simulink model "Traffic_Light_cs - 原始版本留存"  (R2020a)
settings: Solver=ode5  StartTime=0.0  StopTime=200  FixedStep=1/1000  RelTol=1e-3
PreLoadFcn:
  | mbxruntime.callbacks.PreLoadFcn(bdroot);
PostLoadFcn:
  | mbxruntime.callbacks.PostLoadFcn(bdroot);
InitFcn:
  | mbxruntime.callbacks.InitFcn(bdroot);
StartFcn:
  | mbxruntime.callbacks.StartFcn(bdroot);
StopFcn:
  | mbxruntime.callbacks.StopFcn(bdroot);
model workspace (MAT data in the model file):
  mbox_table : object (value not decoded)
  model_closed = 0
  sim_status = 0
values from neighbouring files (symbols this model uses):
  q_pass = [0 0 0 37.0489514481 49.8894252687 51.0913174965 61.791576133 65.4762304223 75.669686677 80.4628164105 88.6197377629 94.2384891559 ... (437675 elements, 87535x5)]    [Data_ckx.mat]
  q_stop = [0 0 0 15.0544571491 15.7911831418 16.0935138936 18.6666396431 19.4721381181 21.7098800606 22.5642135149 25.0883481215 26.1253405703 ... (437675 elements, 87535x5)]    [Data_ckx.mat]
  s = roadinf.s    [Constraint_T_V.m]    (also in Light_Distinguish_old.m = 75:-0.7:75-84*0.7)
undefined symbols (not defined in the file or in its folder): InitImageOutputDir, mbxruntime, sigbuilder_block, tabledata
libraries: simulink x10, PreScanSimulinkLibrary x8, simulink_extras x4, autolibshared x1, fuzblock x1
(part 5 of 5)

== matlab function Traffic_Light_cs - 原始版本留存/CAR_Ahead/Decision/Function-Call Subsystem/Subsystem/MATLAB Function ==
  data: Dis input; R_Ori input; Light_State output; G_Ori input; B_Ori input
function Light_State = Light_Distinguish(Dis,R_Ori,G_Ori,B_Ori)

Image=zeros(1800,1920,3);

Image(:,:,1)=R_Ori;
Image(:,:,2)=G_Ori;
Image(:,:,3)=B_Ori;

Light_State=-1;

if Dis>=75
    Light_State=-1;
else
    %%
    
    Gray=rgb2gray(Image);
    
    R=Image(:,:,1); G=Image(:,:,2); B=Image(:,:,3);
    % figure(1),
    % subplot(2,2,1),imshow(Image),title('image')
    % subplot(2,2,2),imshow(R),title('r')
    % subplot(2,2,3),imshow(G),title('g')
    % subplot(2,2,4),imshow(B),title('b')
    
    diff_R=80; diff_G=30; diff_B=10;  % 设置红、绿、蓝三种颜色提取阈值（越大越严格）
    s=75:-0.7:75-84*0.7;
    yy=[765 762 760 759 758 756 755 753 751 750 748 746 744 743 742 740 738 737 734 732 731 729 ...
     727 725 722 720 718 716 712 711 707 705 702 700 695 694 690 687 682 680 678 671 670 666 ...
     663 656 653 650 646 640 636 631 627 621 616 608 602 597 592 587 577 570 562 551 544 536 528 ...
     516 505 495 483 473 459 443 429 413 395 379 358 336 312 289 262 242 202];
    p=polyfit(s,yy,5);
    start=ceil(polyval(p,Dis));
    start=max(start-50,1);     %搜索窗上限
    %%
    % 红色提取
    
    Image_R=Image;
    
    RP_R=Image(:,:,1); RP_G=Image(:,:,2); RP_B=Image(:,:,3);
    
    % figure(2),
    % subplot(2,2,1),imshow(Image),title('image')
    % subplot(2,2,2),imshow(RP_R),title('RP_Rr')
    % subplot(2,2,3),imshow(RP_G),title('RP_Gg')
    % subplot(2,2,4),imshow(RP_B),title('RP_Bb')
    
    XYR=~((R-G)>diff_R&(R-B)>diff_R);  % 提取红色条件是R分量与G、B分量差值大于设定
    
    Mask=Gray(XYR);  % 灰照片掩膜
    
    RP_R(XYR)=Mask; RP_G(XYR)=Mask; RP_B(XYR)=Mask;  % 使得非红色区域变为灰色
    
    Image_R(:,:,1)=RP_R; Image_R(:,:,2)=RP_G; Image_R(:,:,3)=RP_B;
    if start<=300
        start=310;
    end
    SearchRangeR=XYR(start-300:start+200,700:1240);   %确定搜索范围
    if length(find((SearchRangeR)==0))>=1
        Light_State=1;
    end
    
    %%
    % 绿色提取
    Image_G=Image;
    
    GP_R=Image(:,:,1); GP_G=Image(:,:,2); GP_B=Image(:,:,3);
    
    XYG=~((G-R)>diff_G&(G-B)>diff_G);  % 提取绿色条件是G分量与R、B分量差值大于设定
    
    % Mask=Gray(XYG);  % 灰照片掩膜
    Mask=0;
    
    GP_R(XYG)=Mask; GP_G(XYG)=Mask; GP_B(XYG)=Mask;  % 使得非绿色区域变为灰色
    
    Image_G(:,:,1)=GP_R; Image_G(:,:,2)=GP_G; Image_G(:,:,3)=GP_B;
    
    if start<=100
        start=110;
    end
    SearchRangeG=XYG(start-100:start+200,500:1420);   %确定搜索范围
    
    if length(find((SearchRangeG)==0))>=50
        Light_State=2;
    end
    
    %%
    % 蓝色提取
    
    Image_B=Image;
    
    BP_R=Image(:,:,1);BP_G=Image(:,:,2);BP_B=Image(:,:,3);
    
    XYB=~((B-R)>diff_B&(B-G)>diff_B);  % 提取绿色条件是G分量与R、B分量差值大于设定
    
    Mask_B=Gray(XYB);  % 灰照片掩膜
    
    BP_R(XYB)=Mask_B; BP_G(XYB)=Mask_B; BP_B(XYB)=Mask_B;  % 使得非蓝色区域变为灰色
    
    Image_B(:,:,1)=BP_R; Image_B(:,:,2)=BP_G; Image_B(:,:,3)=BP_B;
    
    %%
%     显示结果
%     figure
%     subplot(2,2,1),imshow(Image); title('Image');
%     
%     subplot(2,2,2),imshow(Image_R); title('Red Pass');
%     
%     subplot(2,2,3),imshow(Image_G); title('Green Pass');
%     
%     subplot(2,2,4),imshow(Image_B); title('Blue Pass');
%     
%     figure,
%     subplot(1,2,1),imshow(Image); title('Image');
%     subplot(1,2,2),imshow(Image_G); title('Green Pass');
%     显示原图与R/G/B三色提取结果对比图并显示标签
end
end

== matlab function Traffic_Light_cs - 原始版本留存/CAR_Ahead/Subsystem/MATLAB Function ==
  data: Car_GPS input; TrafficLight_GPS input; TrafficLight_ID output; Dis_Car2Light output
function [TrafficLight_ID,Dis_Car2Light] = fcn(Car_GPS, TrafficLight_GPS)

Car_X=Car_GPS(2);
Car_Xdelay=Car_GPS(1);
deltax=(Car_X-Car_Xdelay);
if deltax==0
    deltax = 0.001;
end

Car_Y=Car_GPS(4);
Car_Ydelay=Car_GPS(3);
deltay=(Car_Y-Car_Ydelay);
if deltay==0
    deltay = 0.001;
end

TrafficLight_ID=0;
Dis_Car2Light=inf;
Ang_Car2Light=-inf;
Index_Car2Light=-inf;

x1=[deltax,deltay];

for ID=1:3
    Dx=-Car_X+TrafficLight_GPS(2*ID-1);
    Dy=-Car_Y+TrafficLight_GPS(2*ID);
    x2=[Dx,Dy];
    Ang=dot(x1,x2)/(norm(x1)*norm(x2));
    Dis=norm(x2);
    if Dis==0
        Dis=0.001;
    end
    Index=Ang/(Dis)^0.2;
    if Index>Index_Car2Light
        TrafficLight_ID=ID;
        Dis_Car2Light=norm(x2);
        Index_Car2Light=Index;
    end
end

== matlab function Traffic_Light_cs - 原始版本留存/CAR_Main/Decision/Function-Call Subsystem/Speed Decision by Q_leaning/MATLAB Function2 ==
  data: dis input; index_p output; vnow input
function index_p = index_pass(dis,vnow)

index_p=((500-dis)/0.2)*35+(vnow-5.6)/0.4+1;

== matlab function Traffic_Light_cs - 原始版本留存/CAR_Main/Decision/Function-Call Subsystem/Speed Decision by Q_leaning/MATLAB Function3 ==
  data: u1 input; a output; u2 input; u3 input; u4 input; u5 input
function a = a_cal(u1,u2,u3,u4,u5)
max=0;
s=0;
if u1>max
    max = u1;
    s=-1.2;
end
if u2>max
    max = u2;
    s=-0.4;
end
if u3>max
    max = u3;
    s=0;
end
if u4>max
    max = u4;
    s=0.4;
end
if u5>max
    max = u5;
    s=1.2;
end
a=s;

== stateflow chart Traffic_Light_cs - 原始版本留存/ID_1/Traffic Light Logic  ==
  state Initial
    en:
    RedState=0;
    GreenState=1;
    YellowState=0;
    PhaseTime= 51;
  state RedLight
    en,du:
    RedState=1;
    GreenState=0;
    YellowState=0;
  state YellowLight
    en,du:
    RedState=0;
    GreenState=0;
    YellowState=1;
  state GreenLight
    en,du:
    RedState=0;
    GreenState=1;
    YellowState=0;
  (default) -> Initial
  Initial -> YellowLight [order 2] : [YellowState==1&&PhaseTime<=3]
  Initial -> GreenLight [order 3] : [GreenState==1&&PhaseTime<=56]
  Initial -> RedLight [order 1] : [RedState==1&&PhaseTime<=62]
  YellowLight -> YellowLight [order 2] : [PhaseTime>0]
      | {PhaseTime=PhaseTime-0.001;}
  RedLight -> RedLight [order 2] : [PhaseTime>0]
      | {PhaseTime=PhaseTime-0.001;}
  YellowLight -> RedLight [order 1] : [PhaseTime<=0]
      | {PhaseTime= 62;}
  RedLight -> GreenLight [order 1] : [PhaseTime<=0]
      | {PhaseTime= 56;}
  GreenLight -> YellowLight [order 1] : [PhaseTime<=0]{PhaseTime=3;}
  GreenLight -> GreenLight [order 2] : [PhaseTime>0]
      | {PhaseTime=PhaseTime-0.001;}
  data: GreenState output double; YellowState output double; RedState output double; PhaseTime output double; Time input double

== matlab function Traffic_Light_cs - 原始版本留存/CAR_Main/Decision/Function-Call Subsystem/Speed Decision by Q_leaning/MATLAB Function4 ==
  data: dis input; index_s output; vnow input
function index_s  = index_stop(dis,vnow)

dis_n = ceil(dis/0.2)*0.2;
vnow_n = ceil(vnow/0.4)*0.4;

a = (500-dis_n)*175;
b = (vnow_n-0.4)/0.4;

index_s = a+b+1;

== stateflow chart Traffic_Light_cs - 原始版本留存/ID_2/Traffic Light Logic  ==
  state Initial
    en:
    RedState=0;
    GreenState=0;
    YellowState=0;
    PhaseTime= 0;
  state RedLight
    en,du:
    RedState=1;
    GreenState=0;
    YellowState=0;
  state YellowLight
    en,du:
    RedState=0;
    GreenState=0;
    YellowState=1;
  state GreenLight
    en,du:
    RedState=0;
    GreenState=1;
    YellowState=0;
  (default) -> Initial
  Initial -> RedLight : [PhaseTime<=0]{PhaseTime= 62;}
  YellowLight -> YellowLight [order 2] : [PhaseTime>0]
      | {PhaseTime=PhaseTime-0.001;}
  RedLight -> RedLight [order 2] : [PhaseTime>0]
      | {PhaseTime=PhaseTime-0.001;}
  YellowLight -> RedLight [order 1] : [PhaseTime<=0]
      | {PhaseTime= 62;}
  RedLight -> GreenLight [order 1] : [PhaseTime<=0]
      | {PhaseTime= 56;}
  GreenLight -> YellowLight [order 1] : [PhaseTime<=0]{PhaseTime=3;}
  GreenLight -> GreenLight [order 2] : [PhaseTime>0]
      | {PhaseTime=PhaseTime-0.001;}
  data: GreenState output double; YellowState output double; RedState output double; PhaseTime output double; Time input double

== stateflow chart Traffic_Light_cs - 原始版本留存/ID_3/Traffic Light Logic  ==
  state Initial
    en:
    RedState=0;
    GreenState=0;
    YellowState=0;
    PhaseTime= 0;
  state RedLight
    en,du:
    RedState=1;
    GreenState=0;
    YellowState=0;
  state YellowLight
    en,du:
    RedState=0;
    GreenState=0;
    YellowState=1;
  state GreenLight
    en,du:
    RedState=0;
    GreenState=1;
    YellowState=0;
  (default) -> Initial
  Initial -> RedLight : [PhaseTime<=0]{PhaseTime= 62;}
  YellowLight -> YellowLight [order 2] : [PhaseTime>0]
      | {PhaseTime=PhaseTime-0.001;}
  RedLight -> RedLight [order 2] : [PhaseTime>0]
      | {PhaseTime=PhaseTime-0.001;}
  YellowLight -> RedLight [order 1] : [PhaseTime<=0]
      | {PhaseTime= 62;}
  RedLight -> GreenLight [order 1] : [PhaseTime<=0]
      | {PhaseTime= 56;}
  GreenLight -> YellowLight [order 1] : [PhaseTime<=0]{PhaseTime=3;}
  GreenLight -> GreenLight [order 2] : [PhaseTime>0]
      | {PhaseTime=PhaseTime-0.001;}
  data: GreenState output double; YellowState output double; RedState output double; PhaseTime output double; Time input double

== stateflow chart Traffic_Light_cs - 原始版本留存/CAR_Main/Decision/Function-Call Subsystem/Speed Decision by Q_leaning/Chart ==
  state Initial
    en:
    V_local = V_now;
  state Phase_a
    en:
    V_target = V_local;
    V_local = V_target;
    du:
    count  = count-1;
  state Phase_a1
    en:
    count = 2;
    V_target = V_local+Acc;
    du:
    count  = count-1;
  (default) -> Initial
  Initial -> Phase_a1
  Phase_a -> Phase_a1 : [count == 0]{count = 2;}
  Phase_a1 -> Phase_a : [count == 0]
      | {count = 2;}
  data: Acc input; V_now input; V_target output; count local; count2 local; V_local output

== stateflow chart Traffic_Light_cs - 原始版本留存/CAR_Main/Decision/Function-Call Subsystem/Speed Decision by Q_leaning/Memory ==
  state Initial
    en:
    V_target = Original;
    count = 50;
  state Mem
    du:
    count = count - 1;
  (default) -> Initial
  Initial -> Mem : [count>0]
  Mem -> Initial : [count<=0]
  data: Original input; V_target output; count local

== stateflow chart Traffic_Light_cs - 原始版本留存/CAR_Main/Decision/Function-Call Subsystem/Speed Decision by Q_leaning/Memory2 ==
  state Initial
    en:
    V_target = Original;
    count = 50;
  state Mem
    du:
    count = count - 1;
  (default) -> Initial
  Initial -> Mem : [count>0]
  Mem -> Initial : [count<=0]
  data: Original input; V_target output; count local

== matlab function Traffic_Light_cs - 原始版本留存/CAR_Main/Subsystem/MATLAB Function ==
  data: Car_GPS input; TrafficLight_GPS input; TrafficLight_ID output; Dis_Car2Light output
function [TrafficLight_ID,Dis_Car2Light] = fcn(Car_GPS, TrafficLight_GPS)

Car_X=Car_GPS(2);
Car_Xdelay=Car_GPS(1);
deltax=(Car_X-Car_Xdelay);
if deltax==0
    deltax = 0.001;
end

Car_Y=Car_GPS(4);
Car_Ydelay=Car_GPS(3);
deltay=(Car_Y-Car_Ydelay);
if deltay==0
    deltay = 0.001;
end

TrafficLight_ID=0;
Dis_Car2Light=inf;
Ang_Car2Light=-inf;
Index_Car2Light=-inf;

x1=[deltax,deltay];

for ID=1:3
    Dx=-Car_X+TrafficLight_GPS(2*ID-1);
    Dy=-Car_Y+TrafficLight_GPS(2*ID);
    x2=[Dx,Dy];
    Ang=dot(x1,x2)/(norm(x1)*norm(x2));
    Dis=norm(x2);
    if Dis==0
        Dis=0.001;
    end
    Index=Ang/(Dis)^0.2;
    if Index>Index_Car2Light
        TrafficLight_ID=ID;
        Dis_Car2Light=norm(x2);
        Index_Car2Light=Index;
    end
end

== matlab function Traffic_Light_cs - 原始版本留存/CAR_Main/Decision/Function-Call Subsystem/Subsystem/MATLAB Function ==
  data: Dis input; R_Ori input; Light_State output; G_Ori input; B_Ori input
function Light_State = Light_Distinguish(Dis,R_Ori,G_Ori,B_Ori)

Image=zeros(1800,1920,3);

Image(:,:,1)=R_Ori;
Image(:,:,2)=G_Ori;
Image(:,:,3)=B_Ori;

Light_State=-1;

if Dis>=75
    Light_State=-1;
else
    %%
    
    Gray=rgb2gray(Image);
    
    R=Image(:,:,1); G=Image(:,:,2); B=Image(:,:,3);
    % figure(1),
    % subplot(2,2,1),imshow(Image),title('image')
    % subplot(2,2,2),imshow(R),title('r')
    % subplot(2,2,3),imshow(G),title('g')
    % subplot(2,2,4),imshow(B),title('b')
    
    diff_R=80; diff_G=30; diff_B=10;  % 设置红、绿、蓝三种颜色提取阈值（越大越严格）
    s=75:-0.7:75-84*0.7;
    yy=[765 762 760 759 758 756 755 753 751 750 748 746 744 743 742 740 738 737 734 732 731 729 ...
        727 725 722 720 718 716 712 711 707 705 702 700 695 694 690 687 682 680 678 671 670 666 ...
        663 656 653 650 646 640 636 631 627 621 616 608 602 597 592 587 577 570 562 551 544 536 528 ...
        516 505 495 483 473 459 443 429 413 395 379 358 336 312 289 262 242 202];
    p=polyfit(s,yy,5);
    start=ceil(polyval(p,Dis));
    start=max(start-50,1);     %搜索窗上限
    %%
    % 红色提取
    
    Image_R=Image;
    
    RP_R=Image(:,:,1); RP_G=Image(:,:,2); RP_B=Image(:,:,3);
    
    % figure(2),
    % subplot(2,2,1),imshow(Image),title('image')
    % subplot(2,2,2),imshow(RP_R),title('RP_Rr')
    % subplot(2,2,3),imshow(RP_G),title('RP_Gg')
    % subplot(2,2,4),imshow(RP_B),title('RP_Bb')
    
    XYR=~((R-G)>diff_R&(R-B)>diff_R);  % 提取红色条件是R分量与G、B分量差值大于设定
    
    Mask=Gray(XYR);  % 灰照片掩膜
    
    RP_R(XYR)=Mask; RP_G(XYR)=Mask; RP_B(XYR)=Mask;  % 使得非红色区域变为灰色
    
    Image_R(:,:,1)=RP_R; Image_R(:,:,2)=RP_G; Image_R(:,:,3)=RP_B;
    if start<=300
        start=310;
    end
    SearchRangeR=XYR(start-300:start+200,300:1620);   %确定搜索范围
    
    if length(find((SearchRangeR)==0))>=50
        Light_State=1;
    end
    
    %%
    % 绿色提取
    Image_G=Image;
    
    GP_R=Image(:,:,1); GP_G=Image(:,:,2); GP_B=Image(:,:,3);
    
    XYG=~((G-R)>diff_G&(G-B)>diff_G);  % 提取绿色条件是G分量与R、B分量差值大于设定
    
    % Mask=Gray(XYG);  % 灰照片掩膜
    Mask=0;
    
    GP_R(XYG)=Mask; GP_G(XYG)=Mask; GP_B(XYG)=Mask;  % 使得非绿色区域变为灰色
    
    Image_G(:,:,1)=GP_R; Image_G(:,:,2)=GP_G; Image_G(:,:,3)=GP_B;
    
    if start<=100
        start=110;
    end
    SearchRangeG=XYG(start-100:start+200,500:1420);   %确定搜索范围
    
    if length(find((SearchRangeG)==0))>=50
        Light_State=2;
    end
    
    %%
    % 蓝色提取
    
    Image_B=Image;
    
    BP_R=Image(:,:,1);BP_G=Image(:,:,2);BP_B=Image(:,:,3);
    
    XYB=~((B-R)>diff_B&(B-G)>diff_B);  % 提取绿色条件是G分量与R、B分量差值大于设定
    
    Mask_B=Gray(XYB);  % 灰照片掩膜
    
    BP_R(XYB)=Mask_B; BP_G(XYB)=Mask_B; BP_B(XYB)=Mask_B;  % 使得非蓝色区域变为灰色
    
    Image_B(:,:,1)=BP_R; Image_B(:,:,2)=BP_G; Image_B(:,:,3)=BP_B;
    
    %%
    % 显示结果
    % figure
    % subplot(2,2,1),imshow(Image); title('Image');
    %
    % subplot(2,2,2),imshow(Image_R); title('Red Pass');
    %
    % subplot(2,2,3),imshow(Image_G); title('Green Pass');
    
    % subplot(2,2,4),imshow(Image_B); title('Blue Pass');
    
    % figure,
    % subplot(1,2,1),imshow(Image); title('Image');
    % subplot(1,2,2),imshow(Image_G); title('Green Pass');
    % 显示原图与R/G/B三色提取结果对比图并显示标签
end
end

== stateflow chart Traffic_Light_cs - 原始版本留存/CAR_Main/Decision/Chart ==
  state Initial_State
  state Decision_State
  (default) -> Initial_State
  Initial_State -> Decision_State : [Dis_Car2Light_0919_100<=500]{Decision_Call;}
  Decision_State -> Initial_State [order 2]
  Decision_State -> Initial_State [order 1] : [Dis_Car2Light_0919_100>500]
  data: Dis_Car2Light_0919_100 input
  events: Decision_Call output FUNCTION_CALL_EVENT

== matlab function Traffic_Light_cs - 原始版本留存/CAR_Main/V2V_Input/MATLAB Function ==
  data: Traffic_ID input; TrafficLight_ID_Ahead input; Light_State_Ahead input; Traffic_Time1 input; Traffic_now_State output; Traffic_now_Time output; Traffic_next_State output; Traffic_next_Time output; TrafficID_Next input; State_Next input; Time_Next input
function [Traffic_now_State,Traffic_now_Time,Traffic_next_State,Traffic_next_Time] = fcn(Traffic_ID,TrafficLight_ID_Ahead,Light_State_Ahead,Traffic_Time1,TrafficID_Next, State_Next, Time_Next)
%% 初始化
% TrafficLight_ID_069_100,Light_State_069_100,Traffic_Time2, 

Traffic_now_State=-1;
Traffic_now_Time=-1;


Traffic_next_State=-1;
Traffic_next_Time=-1;

NextTrafficID=Traffic_ID+1;

%% 存储当前信号灯的状态
if(Traffic_ID==TrafficLight_ID_Ahead)
        Traffic_now_State = Light_State_Ahead;
        Traffic_now_Time = Traffic_Time1;
    
end
%% 存储下一个信号灯的状态
if(NextTrafficID==TrafficLight_ID_Ahead)
        Traffic_next_State = Light_State_Ahead;
        Traffic_next_Time = Traffic_Time1;
end
%% 检查有无下一信号灯的存储信息（也就是在第一个灯前面，有没有第二个灯的信息被记录）
if Traffic_ID==TrafficID_Next
    Traffic_now_State = State_Next;
    Traffic_now_Time = Time_Next;
end


end

== stateflow chart Traffic_Light_cs - 原始版本留存/CAR_Main/V2V_Input/Chart1 ==
  state Initial
    en:
    state=-1;
    time=-1;
    du:
    localID=TrafficID;
  state GetInformation
    en:
    local_state=now_state;
    local_time=now_time;
  state Green
  state Yellow
  state Red
  state delay
    en:
    countdelay = 1000;
    du:
    countdelay =countdelay - 1;
  (default) -> Initial
  delay -> Initial [order 4] : [countdelay<=0]
  Initial -> GetInformation : [now_state>0]{localID=TrafficID;}
  GetInformation -> Red [order 1] : [local_state==1]
      | {time=local_time;state=local_state;}
  GetInformation -> Yellow [order 3] : [local_state==0]
      | {time=local_time;state=local_state;}
  GetInformation -> Green [order 2] : [local_state==2]
      | {time=local_time;state=local_state;}
  Green -> Green [order 3] : [time>0]
      | {time=time-0.001;}
  Green -> Yellow [order 2] : [time<=0]
      | {time=3;state=0;}
  delay -> Green [order 3] : [localID==TrafficID]
  Green -> delay [order 1] : [localID~=TrafficID]
  Red -> Green [order 1] : [time<=0]
      | {time=56;state=2;}
  Red -> Red [order 2] : [time>0]
      | {time=time-0.001;}
  Yellow -> Yellow [order 2] : [time>0]
      | {time=time-0.001;}
  delay -> Yellow [order 1] : [localID==TrafficID]
  Yellow -> delay [order 3] : [localID~=TrafficID]
  Yellow -> Red [order 1] : [time<=0]
      | {time=62;
      | state=1;}
  delay -> Red [order 2] : [localID==TrafficID]
  Red -> delay [order 3] : [localID~=TrafficID]
  data: TrafficID input; now_state input; now_time input; state output; time output; local_state local; local_time local; localID local; countdelay local

== stateflow chart Traffic_Light_cs - 原始版本留存/CAR_Main/V2V_Input/Chart2 ==
  state Initial
    en:
    state=-1;
    time=-1;
    du:
    localnextID=TrafficID+1;
  state delay
    en:
    countdelay = 2000;
    du:
    countdelay =countdelay - 1;
  state GetInformation
    en:
    local_state=next_state;
    local_time=next_time;
  state Green
  state Yellow
  state Red
  (default) -> Initial
  Initial -> delay : [next_state>0]
  delay -> Initial [order 2] : [countdelay<=0]
  delay -> Red [order 5] : [localnextID==TrafficID+1&&state==1]
  Yellow -> delay [order 2] : [localnextID~=TrafficID+1]
  delay -> Yellow [order 3] : [localnextID==TrafficID+1&&state==0]
  Red -> delay [order 1] : [localnextID~=TrafficID+1]
  Green -> delay [order 2] : [localnextID~=TrafficID+1]
  delay -> Green [order 4] : [localnextID==TrafficID+1&&state==2]
  delay -> GetInformation [order 1] : [next_state>0&&countdelay<=0]
  GetInformation -> Red [order 1] : [local_state==1]
      | {time=local_time;;state=local_state;}
  GetInformation -> Yellow [order 3] : [local_state==0]
      | {time=local_time;state=local_state;}
  GetInformation -> Green [order 2] : [local_state==2]
      | {time=local_time;state=local_state;}
  Green -> Green [order 3] : [time>0]
      | {time=time-0.001}
  Green -> Yellow [order 1] : [time<=0]
      | {time=3;
      | state=0;}
  Red -> Green [order 2] : [time<=0]
      | {time=56;
      | state=2;}
  Yellow -> Yellow [order 3] : [time>0]
      | {time=time-0.001}
  Red -> Red [order 3] : [time>0]
      | {time=time-0.001}
  Yellow -> Red [order 1] : [time<=0]
      | {time=62;
      | state=1;}
  data: TrafficID input; next_state input; next_time input; state output; time output; local_state local; local_time local; localnextID output; countdelay local

== stateflow chart Traffic_Light_cs - 原始版本留存/CAR_Main/Decision/Function-Call Subsystem/Chart ==
  state Initial
  state Camera
  (default) -> Initial
  Camera -> Initial
  Initial -> Camera : [Traffic_State<0]
      | {Camera_Call;
      | }
  data: Traffic_State input
  events: Camera_Call output FUNCTION_CALL_EVENT

== matlab function Traffic_Light_cs - 原始版本留存/CAR_Main/Decision/Function-Call Subsystem/MATLAB Function ==
  data: lighttype input; tmin output; vehicle_num input; lighttime input; s input; tmax output; suggest output; suggest_delay input
function [tmin,tmax,suggest] = Constraint_T_V(lighttype,vehicle_num,lighttime,s, suggest_delay)
tmin=-1;
tmax=-1;
suggest=-1;
if lighttype<2&&suggest_delay==4
    suggest=4;
else
    Vmax=70/3.6;
    Vmin=20/3.6;
    redtime=62;
    greentime=56;
    yellowtime=3;
    velocity=0.8;
    t_loss=1.5;
    if lighttype >0
        if lighttype==2
            if s/Vmax<lighttime
                tmin=s/Vmax;
                tmax=lighttime;
                suggest=1;    %当前相位通过交叉路口
            elseif redtime+yellowtime+lighttime>=s/Vmin
                tmin=0;
                tmax=0;
                suggest=4;      %停车等待
            % elseif redtime+yellowtime+lighttime<s/Vmin
            %    tmin=redtime+yellowtime+lighttime;
            %    tmax=s/Vmin;
            %    suggest=2;     %考虑在下一个相位通过交叉路口
            end
        else
            if lighttype==0
                lighttime=lighttime+redtime;
            end
            if s/Vmin<=lighttime+vehicle_num/velocity+t_loss
                tmin=0;
                tmax=0;
                suggest=4;      %停车等待
            else
                tmin=lighttime+vehicle_num/velocity+t_loss;
                tmax=s/Vmin;
                suggest=3;     %等待红灯过去，的下一个绿灯范围内通过
            end
        end
    end
end
end

== stateflow chart Traffic_Light_cs - 原始版本留存/CAR_Main/Decision/Function-Call Subsystem/Subsystem/Delay ==
  state Initial
    en:
    Local_State=Light_State_0919_100;
    count1=500;
  state Delay
    en:
    Light_State_End=Local_State;
  (default) -> Initial
  Initial -> Delay : [count1>0]
  Delay -> Initial [order 1] : [count1<=0]
  Delay -> Delay [order 3] : [Local_State~=Light_State_0919_100&&Light_State_0919_100==-1]
      | {count1=count1-1;}
  Delay -> Delay [order 2] : [Local_State~=Light_State_0919_100&&Light_State_0919_100>=0]
      | {count1=0;}
  data: Light_State_0919_100 input; Light_State_End output; Local_State local; count1 local

== stateflow chart Traffic_Light_cs - 原始版本留存/CAR_Ahead/Decision/Chart ==
  state Initial_State
  state Decision_State
  (default) -> Initial_State
  Initial_State -> Decision_State : [Dis_Car2Light_0919_100<=500]{Decision_Call;}
  Decision_State -> Initial_State [order 2]
  Decision_State -> Initial_State [order 1] : [Dis_Car2Light_0919_100>500]
  data: Dis_Car2Light_0919_100 input
  events: Decision_Call output FUNCTION_CALL_EVENT

== stateflow chart Traffic_Light_cs - 原始版本留存/CAR_Ahead/Decision/Function-Call Subsystem/Chart ==
  state Initial
  state Camera
  (default) -> Initial
  Camera -> Initial
  Initial -> Camera : [Traffic_State<0]
      | {Camera_Call;
      | }
  data: Traffic_State input
  events: Camera_Call output FUNCTION_CALL_EVENT

== matlab function Traffic_Light_cs - 原始版本留存/CAR_Main/Decision/Function-Call Subsystem/Speed Decision by Q_leaning/MATLAB Function1 ==
  data: u1 input; a output; u2 input; u3 input; u4 input; u5 input
function a = a_cal(u1,u2,u3,u4,u5)
max=0;
s=0;
if u1>max
    max = u1;
    s=-1.2;
end
if u2>max
    max = u2;
    s=-0.4;
end
if u3>max
    max = u3;
    s=0;
end
if u4>max
    max = u4;
    s=0.4;
end
if u5>max
    max = u5;
    s=1.2;
end
a=s;
